simulink model "magnetic_pendulum"  (R2024b)
settings: Solver=ode45  StartTime=0.0  StopTime=15.0  MaxStep=0.02  MinStep=0.01  RelTol=1e-3
settings Model: Creator=zv53855  LastModifiedBy=zv53855
settings SolverCC: InitialStep=0.01

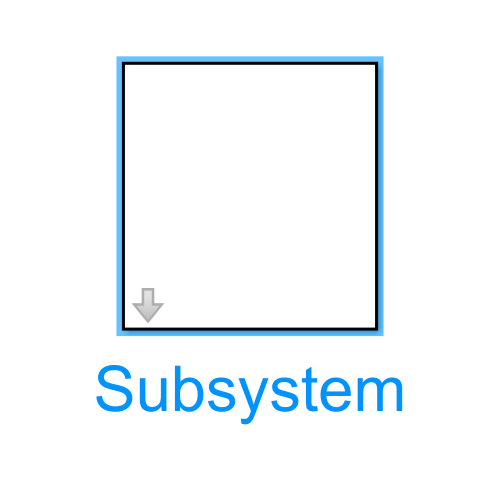
[thumbnail: Simulink's stored preview of the top-level diagram]
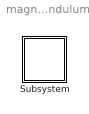
== system magnetic_pendulum ==
  Subsystem : Subsystem  mask{n=3, g=9.81, k=1, m=2, l=4, x=-1, y=-1, x_i=[-1 1 1], y_i=[1 1 -1], d_i=[0.1 0.1 0.1], a_i=[1 -1 1.5]}
      mask prompts: n "magnets num"; g "gravity"; k "damping"; m "pendulum mass"; l "pendulum line"; x "starting x (pednulum)"; y "starting y (pendulum)"; x_i "x magnets positions"; y_i "y magnets positions"; d_i "magnets distances from xy"; a_i "magnets' effect on the pendulum"

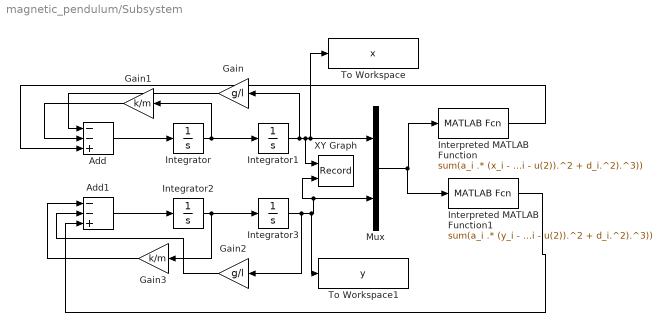
== system magnetic_pendulum/Subsystem ==
  Add : Sum  Inputs=--+
  Add1 : Sum  Inputs=--+
  Gain : Gain  Gain=g/l
  Gain1 : Gain  Gain=k/m
  Gain2 : Gain  Gain=g/l
  Gain3 : Gain  Gain=k/m
  Integrator : Integrator
  Integrator1 : Integrator  InitialCondition=x
  Integrator2 : Integrator
  Integrator3 : Integrator  InitialCondition=y
  Interpreted MATLAB Function : MATLABFcn  MATLABFcn=sum(a_i .* (x_i - u(1)) ./ (sqrt((x_i - u(1)).^2 + (y_i - u(2)).^2 + d_i.^2).^3))
  Interpreted MATLAB Function1 : MATLABFcn  MATLABFcn=sum(a_i .* (y_i - u(2)) ./ (sqrt((x_i - u(1)).^2 + (y_i - u(2)).^2 + d_i.^2).^3))
  Mux : Mux  Inputs=2
  To Workspace : ToWorkspace  VariableName=x  SampleTime=-1
  To Workspace1 : ToWorkspace  VariableName=y  SampleTime=-1
  XY Graph : Record  FileSettingsInternal="{\"entries\":[{\"content\":{\"excelSettings\":{\"content\":{},\"type\":\"Streamout.ExcelSettings\"}},\"type\":\"Streamout.FileSettingStorage\",\"uuid\":\"\"}],\"packageUris\":[\"http:\\/\\/schema.mathworks.com\\/mf0\\/streamout_blocks\\/R2020a\"],\"version\":\"1.0\"}"  Layout=[1 1]  SignalsInternal="{\"entries\":[{\"content\":{\"signals\":[{\"content\":{\"blockPath\":[],\"dimensions\":[1],\"domain\":\"\",\"lineColor\":\"#a2142f\",\"plots\":[ 1 ],\"port\":1,\"sid\":[\"\"],\"signalID\":1,\"signalName\":\"Integrator1\"},\"type\":\"RecordBlkView.Signal\",\"uuid\":\"\"},{\"content\":{\"blockPath\":[],\"dimensions\":[1],\"domain\":\"\",\"lineColor\":\"#139fff\",\"plots\":[ 1 ],\"port\":2,\"sid\":[\"\"],\"signalID\":2,\"signalName\":\"Integrator3\"},\"type\":\"RecordBlkView.Signal\",\"uuid\":\"\"}]},\"type\":\"RecordBlkView.InputSignals\",\"uuid\":\"\"}],\"packageUris\":[\"http:\\/\\/schema.mathworks.com\\/mf0\\/streamout_blocks\\/R2020a\"],\"version\":\"1.0\"}"  VisualizationBindings="{\"xyplotplugin\":{\"info\":[{\"series\":[{\"bindingParametersList\":[{\"parameter\":\"X-Axis\",\"signalID\":1,\"signalName\":\"Integrator1\"},{\"parameter\":\"Y-Axis\",\"signalID\":2,\"signalName\":\"Integrator3\"}],\"seriesID\":0}],\"subplotID\":1}]}}"  CompatibilityTag=XY
  wires:
  Integrator2/1 -> Integrator3/1, Gain3/1
  Integrator/1 -> Integrator1/1, Gain1/1
  Add/1 -> Integrator/1
  Add1/1 -> Integrator2/1
  Integrator3/1 -> Gain2/1, To Workspace1/1, Mux/2, XY Graph/2
  Integrator1/1 -> Gain/1, XY Graph/1, To Workspace/1, Mux/1
  Mux/1 -> Interpreted MATLAB Function1/1, Interpreted MATLAB Function/1
  Interpreted MATLAB Function/1 -> Add/3
  Interpreted MATLAB Function1/1 -> Add1/3
  Gain2/1 -> Add1/2
  Gain3/1 -> Add1/1
  Gain1/1 -> Add/2
  Gain/1 -> Add/1
